simulink model "exampleSaturationProperty"  (Simulink 7.6)
settings: Solver=ode45  StartTime=0.0  StopTime=10.0  RelTol=1e-3
libraries: carnot x4
settings Model: Creator=drhf  LastModifiedBy=drhf

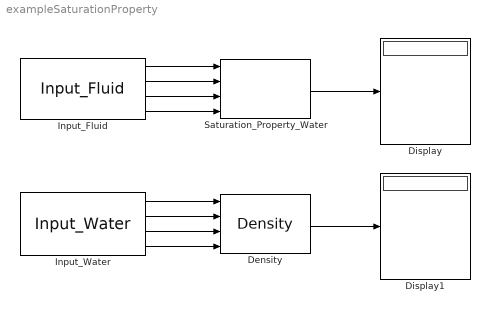
== system exampleSaturationProperty ==
  Density : carnot/Basic/Material_Properties/Density  SystemSampleTime=-1
  Display : Display
  Display1 : Display
  Input_Fluid : carnot/Basic/Material_Properties/Input_Fluid  SystemSampleTime=-1  fluid=water  T=[10:10:50]  p=1e5  x=0.005
  Input_Water : carnot/Basic/Material_Properties/Input_Water  SystemSampleTime=-1  T=[10:10:50]  p=2e6  xd=0
  Saturation_Property_Water : carnot/Basic/Material_Properties/Saturation_Property_Water  SystemSampleTime=-1  prop=density  state=liquid
  wires:
  Input_Fluid/1 -> Saturation_Property_Water/1
  Input_Fluid/2 -> Saturation_Property_Water/2
  Input_Fluid/3 -> Saturation_Property_Water/3
  Input_Fluid/4 -> Saturation_Property_Water/4
  Saturation_Property_Water/1 -> Display/1
  Input_Water/1 -> Density/1
  Input_Water/2 -> Density/2
  Input_Water/3 -> Density/3
  Input_Water/4 -> Density/4
  Density/1 -> Display1/1
